simulink model "FloatShield_PID_Uno"  (R2019a)
settings: Solver=FixedStepDiscrete  StartTime=0.0  StopTime=Inf  FixedStep=0.025  RelTol=1e-3
undefined symbols (not defined in the file): Percentage
libraries: FloatLibrary x1, simulink x1
settings Model: SimulationMode=external  ExtModeTrigDuration=1  Creator=Peter  LastModifiedBy=Peter
settings OptimizationCC: EnhancedBackFolding=on  PassReuseOutputArgsAs=Individual arguments  MaxStackSize=64  OptimizeBlockOrder=speed  DifferentSizesBufferReuse=on  OptimizationCustomize=off
settings DebuggingCC: ParameterTunabilityLossMsg=error
settings HardwareCC: ProdBitPerInt=16  ProdBitPerPointer=16  ProdBitPerSizeT=16  ProdBitPerPtrDiffT=16  ProdLargestAtomicFloat=None  ProdWordSize=8  ProdHWDeviceType=Atmel->AVR
settings SFSimCC: MATLABDynamicMemAlloc=off
settings RTWCC: SystemTargetFile=ert.tlc  HardwareBoard=Arduino Uno  TLCOptions=-aInlineSetEventsForThisBaseRateFcn=TLC_FALSE -aSuppressMultiTaskScheduler=TLC_FALSE -aRateBasedStepFcn=1  TemplateMakefile=ert_default_tmf  GenerateReport=on  Toolchain=Arduino AVR  BuildConfiguration=Faster Runs  IncludeHyperlinkInReport=on  LaunchReport=on  GenerateTraceInfo=on  GenerateTraceReport=on  GenerateTraceReportSl=on  GenerateTraceReportSf=on  GenerateTraceReportEml=on
settings CodeAppCC: ForceParamTrailComments=on  IgnoreCustomStorageClasses=off  OperatorAnnotations=on  SimulinkDataObjDesc=on  SFDataObjDesc=on  InsertBlockDesc=on
settings ERTTargetCC: SupportContinuousTime=on  SupportVariableSizeSignals=on  ExtMode=on  ExtModeStaticAllocSize=250  ExtModeMexArgs='127.0.0.1' 0 17725

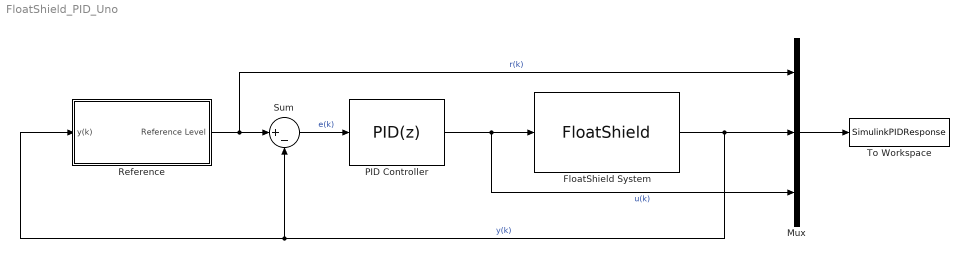
== system FloatShield_PID_Uno ==
  FloatShield System : FloatLibrary/FloatShield  OutRadio=Percentage (%)  Tcal=10  Ts=0.025
      settings: SourceProductName=AutomationShield
  Mux : Mux  Inputs=3
  PID Controller : simulink/Continuous/PID Controller  Controller=PID  Form=Ideal  TimeDomain=Discrete-time  SampleTime=-1  IntegratorMethod=Forward Euler  FilterMethod=Forward Euler  ControllerParametersSource=internal  P=0.25  I=0.2  D=0.01  UseFilter=off  N=100  TunerSelectOption=Transfer Function Based (PID Tuner App)  InitialConditionSource=internal  InitialConditionForIntegrator=0  InitialConditionForFilter=0  DifferentiatorICPrevScaledInput=0  ExternalReset=none  TrackingMode=off  Kt=1  LimitOutput=on  UpperSaturationLimit=100  LowerSaturationLimit=30  LinearizeAsGain=on  AntiWindupMode=none  Kb=1  POutMin=[]  POutMax=[]  IOutMin=[]  IOutMax=[]  DOutMin=[]  DOutMax=[]  NOutMin=[]  NOutMax=[]  SumOutMin=[]  SumOutMax=[]  SaturationOutMin=[]  SaturationOutMax=[]  PParamMin=[]  PParamMax=[]  IParamMin=[]  IParamMax=[]  DParamMin=[]  DParamMax=[]  NParamMin=[]  NParamMax=[]  KbParamMin=[]  KbParamMax=[]  KtParamMin=[]  KtParamMax=[]  KbOutMin=[]  KbOutMax=[]  KtOutMin=[]  KtOutMax=[]  IntegratorOutMin=[]  IntegratorOutMax=[]  FilterOutMin=[]  FilterOutMax=[]  SumI1OutMin=[]  SumI1OutMax=[]  SumI2OutMin=[]  SumI2OutMax=[]  SumI3OutMin=[]  SumI3OutMax=[]  SumI4OutMin=[]  SumI4OutMax=[]  SumDOutMin=[]  SumDOutMax=[]  DifferentiatorOutMin=[]  DifferentiatorOutMax=[]  FilterDiffOutCoefMin=[]  FilterDiffOutCoefMax=[]  ReciprocalOutMin=[]  ReciprocalOutMax=[]  SumDenOutMin=[]  SumDenOutMax=[]  SumNumOutMin=[]  SumNumOutMax=[]  DivideOutMin=[]  DivideOutMax=[]  IntegratorContinuousStateAttributes=''  IntegratorStateMustResolveToSignalObject=off  IntegratorRTWStateStorageClass=Auto  FilterContinuousStateAttributes=''  FilterStateMustResolveToSignalObject=off  FilterRTWStateStorageClass=Auto  ParallelPVariant=Passthrough  IdealPVariant=InternalParameters  IVariant=InternalParameters  DVariant=InternalParameters  IntegratorVariant=Discrete  SatVariant=Enabled  AWVariant=Passthrough  PCopyVariant=Disabled  TRVariant=Disabled  FdbkBlocksVariant=Forward  IdealPFdbkVariant=Disabled  SatFdbkVariant=Disabled  DerivativeFilterVariant=Differentiator  NVariant=Passthrough  NCopyVariant=Disabled_SignalSpec  FilterICVariant=InternalICsDifferentiator  IntegratorICVariant=InternalICs  ExternalResetVariant=Disabled  TRSumVariant=Passthrough  SumFdbkVariant=Disabled  SumVariant=Sum_PID
  Reference : Subsystem  StopFcn=|  mask{RefVect=[65, 50, 35, 45, 60, 75, 55, 40, 20, 30], SectLen=2400, Ts=0.025}
      | if exist('simout')
      | SimulinkPIDResponse=simout;
      | end
      | 
      | if exist('SimulinkPIDResponse')
      | unmodifiedResponse=SimulinkPIDResponse;
      | sectLen = str2num(get_param(strcat(gcs,'/Reference'),'SectLen'));
      | refVect = str2num(get_param(strcat(gcs,'/Reference'),'RefVect'));
      | refLen = length(refVect);
      | responseLen=length(SimulinkPIDResponse(:,1));
      | badSamples = responseLen-sectLen*refLen+1;
      | if badSamples>=1
      | SimulinkPIDResponse=SimulinkPIDResponse(badSamples:end,:);
      | end
      | clear sectLen refVect refLen responseLen badSamples;
      | save SimulinkPIDResponse SimulinkPIDResponse;
      | plotPIDResponse(SimulinkPIDResponse,100);
      | end
      mask prompts: RefVect "Reference Vector:"; SectLen "Section Length (Number of Samples):"; Ts "Sampling Period (s):"
      mask init:
      | CalibTime = str2num(get_param(strcat(gcs,'/FloatShield System'),'Tcal'));
      | CalibTime = round(CalibTime/Ts)*Ts;
      mask DialogControl DescGroupVar Prompt: Reference Block
      mask DialogControl DescTextVar Prompt: Block used to provide changing reference levels during simulation.
  Sum : Sum  Inputs=|+-
  To Workspace : ToWorkspace  VariableName=SimulinkPIDResponse  SampleTime=-1
      settings: Save2DSignal=2-D array (concatenate along first dimension)
  wires:
  PID Controller/1 -> Mux/3, FloatShield System/1  "u(k)"
  Sum/1 -> PID Controller/1  "e(k)"
  Reference/1(Reference Level) -> Mux/1, Sum/1  "r(k)"
  FloatShield System/1 -> Reference/1(y(k)), Sum/2, Mux/2  "y(k)"
  Mux/1 -> To Workspace/1

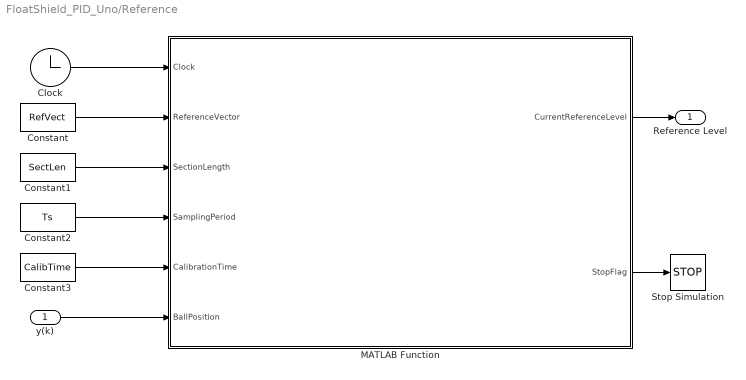
== system FloatShield_PID_Uno/Reference ==
  y(k) : Inport
  Clock : Clock
  Constant : Constant  Value=RefVect  SampleTime=Ts
  Constant1 : Constant  Value=SectLen  SampleTime=Ts
  Constant2 : Constant  Value=Ts  SampleTime=Ts
  Constant3 : Constant  Value=CalibTime  SampleTime=Ts
  MATLAB Function : MATLAB Function  TreatAsAtomicUnit=on
  Stop Simulation : Stop
  Reference Level : Outport
  wires:
  Constant/1 -> MATLAB Function/2(ReferenceVector)
  Constant1/1 -> MATLAB Function/3(SectionLength)
  Constant2/1 -> MATLAB Function/4(SamplingPeriod)
  Clock/1 -> MATLAB Function/1(Clock)
  Constant3/1 -> MATLAB Function/5(CalibrationTime)
  MATLAB Function/1(CurrentReferenceLevel) -> Reference Level/1
  MATLAB Function/2(StopFlag) -> Stop Simulation/1
  y(k)/1 -> MATLAB Function/6(BallPosition)

== matlab function FloatShield_PID_Uno/Reference/MATLAB Function ==
  data: Clock input; CurrentReferenceLevel output; ReferenceVector input; SectionLength input; SamplingPeriod input; StopFlag output; CalibrationTime input; BallPosition input
%     Simulink Block for changing reference train used in PID examples.
%
%     This code is part of the AutomationShield hardware and software
%     ecosystem. Visit http://www.automationshield.com for more
%     details. This code is licensed under a Creative Commons
%     Attribution-NonCommercial 4.0 International License.
%
%     Created by Peter Chmurciak.
%     Last update: 12.8.2019.

function [CurrentReferenceLevel, StopFlag] = fcn(Clock, ReferenceVector, SectionLength, SamplingPeriod, CalibrationTime, BallPosition)

persistent counter liftTime;                            % Persistent variables

if Clock > CalibrationTime                              % Starts after calibration
    if isempty(liftTime)                                % Getting time when ball reaches half value of first reference level
        CurrentReferenceLevel = ReferenceVector(1);
        StopFlag = 0;
        if BallPosition > 0.5 * ReferenceVector(1)
            liftTime = Clock;
        end
    else                                                % Changing reference train
        if isempty(counter)
            counter = 1;
        end
        ReferenceLength = length(ReferenceVector);
        SectionDuration = SectionLength * SamplingPeriod;
        if (Clock - CalibrationTime - liftTime) <= (SectionDuration * counter)
            CurrentReferenceLevel = ReferenceVector(counter);
            StopFlag = 0;
        else
            counter = counter + 1;
            if counter <= ReferenceLength
                CurrentReferenceLevel = ReferenceVector(counter);
                StopFlag = 0;
            else
                CurrentReferenceLevel = ReferenceVector(counter-1);
                StopFlag = 1;                           % Stop simulation at the end of reference train
            end
        end
    end
else
    CurrentReferenceLevel = ReferenceVector(1);
    StopFlag = 0;
end

end                                                     % End of function definition
